simulink model "Matla"  (R2023a)
settings: Solver=VariableStepAuto  StartTime=0.0  StopTime=1/50  RelTol=1e-3
libraries: simulink x1
settings Model: Creator=Hp  LastModifiedBy=Hp

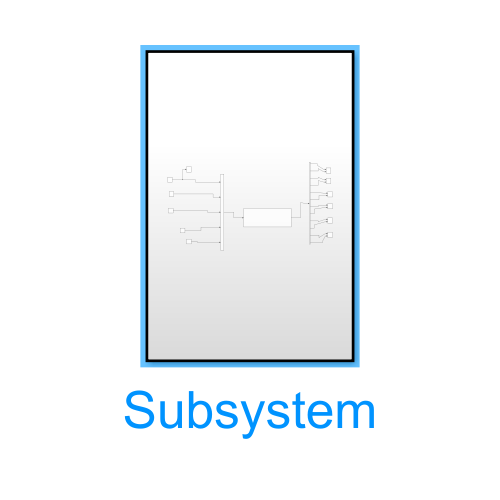
[thumbnail: Simulink's stored preview of the top-level diagram]
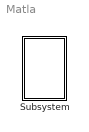
== system Matla ==
  Subsystem : Subsystem

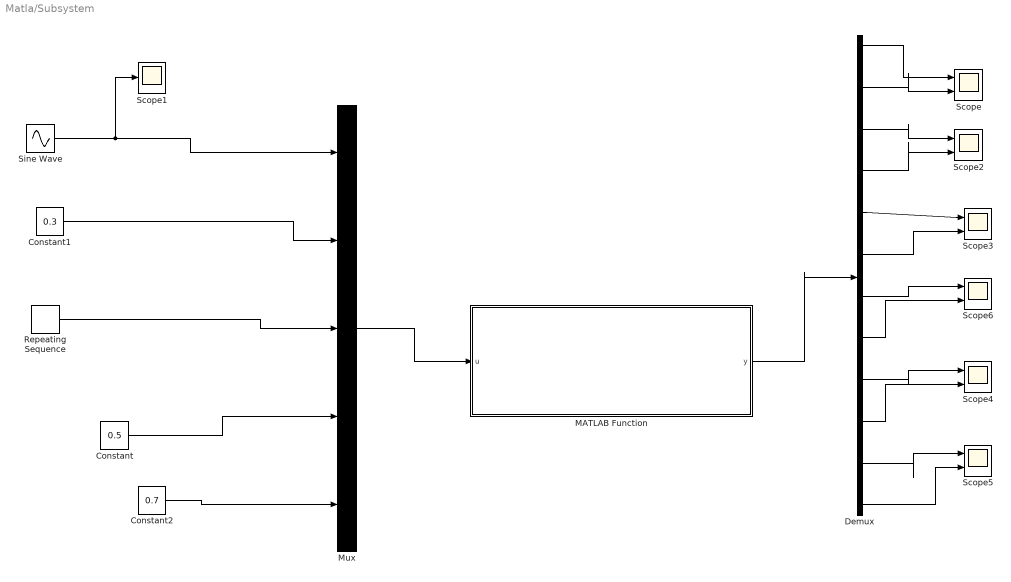
== system Matla/Subsystem ==
  Constant : Constant  Value=0.5
  Constant1 : Constant  Value=0.3
  Constant2 : Constant  Value=0.7
  Demux : Demux  Outputs=12
  MATLAB Function : MATLAB Function  TreatAsAtomicUnit=on
  Mux : Mux  Inputs=5
  Repeating Sequence : simulink/Sources/Repeating Sequence  rep_seq_t=[0 1/25e3]  rep_seq_y=[0 1]
  Scope{,2..6} (6 alike) : Scope  NumInputPorts=2
  Scope1 : Scope
  Sine Wave : Sin  Frequency=2*pi*50  SampleTime=0
  wires:
  Repeating Sequence/1 -> Mux/3
  Demux/11 -> Scope5/1
  Constant/1 -> Mux/4
  Demux/4 -> Scope2/2
  Mux/1 -> MATLAB Function/1(u)
  Demux/3 -> Scope2/1
  Constant2/1 -> Mux/5
  MATLAB Function/1(y) -> Demux/1
  Demux/6 -> Scope3/2
  Demux/7 -> Scope6/1
  Demux/5 -> Scope3/1
  Demux/1 -> Scope/1
  Demux/9 -> Scope4/1
  Demux/8 -> Scope6/2
  Sine Wave/1 -> Mux/1, Scope1/1
  Demux/10 -> Scope4/2
  Constant1/1 -> Mux/2
  Demux/2 -> Scope/2
  Demux/12 -> Scope5/2

== matlab function Matla/Subsystem/MATLAB Function ==
  data: u input; y output
function y = fcn(u)
a=u(1);
b=u(2);
c=u(3);
d=u(4);
e=u(5);
if a>=0
    s1=1;
    s2=0;
    s5=1;
    if(b>=c)
        s3=1;
        s4=0;
    else
        s3=0;
        s4=1;
    end
    s7=0;
    s9=1;
    s11=0;
   
    if(d>=c)
        s8=1;
        s6=0;
    else
        s8=0;
        s6=1;
    end
     if(e>=c)
        s10=1;
        s12=0;
    else
        s10=0;
        s12=1;
    end
else
    s1=0;
    s2=1;
    s5=0;
    s7=1;
    s9=0;
    s11=1;
    if(b>=c)
        s3=0;
        s4=1;
    else
        s3=1;
        s4=0;
    end
    if(d>=c)
        s8=0;
        s6=1;
    else
        s8=1;
        s6=0;
    end
     if(e>=c)
        s10=0;
        s12=1;
    else
        s10=1;
        s12=0;
    end

end
y = [s1;s2;s3;s4;s5;s6;s7;s8;s9;s11;s10;s12];
